simulink model "chap4_3sim"  (Simulink 8.3)
settings: Solver=ode45  StartTime=0.0  StopTime=10.0  RelTol=1e-3
libraries: fuzblock x1
settings Model: Creator=duan  LastModifiedBy=duan
settings DataIOCC: SignalLoggingSaveFormat=Dataset
settings DebuggingCC: UnderspecifiedInitializationDetection=Simplified  StateNameClashWarn=none
settings GRTTargetCC: CombineOutputUpdateFcns=on  GRTInterface=off

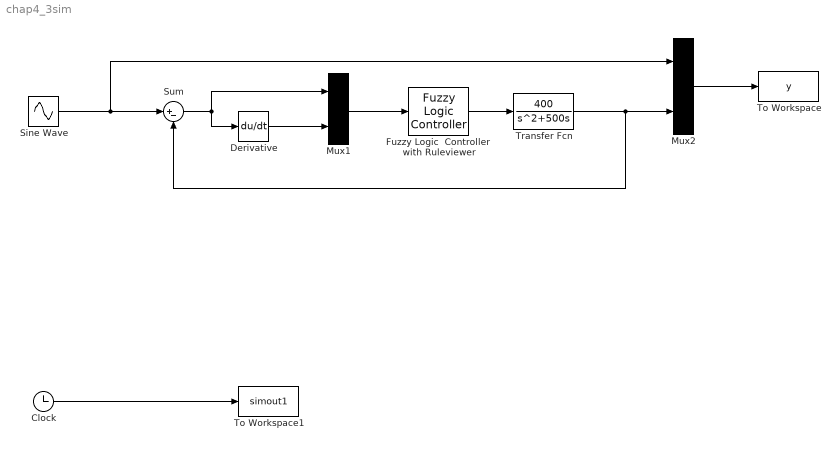
== system chap4_3sim ==
  Clock : Clock
  Derivative : Derivative
  Fuzzy Logic  Controller  with Ruleviewer : fuzblock/Fuzzy Logic  Controller  fis=[]
  Mux1 : Mux  Inputs=2
  Mux2 : Mux  Inputs=2
  Sine Wave : Sin  SampleTime=0
  Sum : Sum  Inputs=|+-
  To Workspace : ToWorkspace  VariableName=y  SaveFormat=Timeseries  SampleTime=-1
  To Workspace1 : ToWorkspace  VariableName=simout1  SaveFormat=Timeseries  SampleTime=-1
  Transfer Fcn : TransferFcn  Numerator=[400]  Denominator=[1 500 0]
  wires:
  Clock/1 -> To Workspace1/1
  Sine Wave/1 -> Mux2/1, Sum/1
  Sum/1 -> Derivative/1, Mux1/1
  Derivative/1 -> Mux1/2
  Mux1/1 -> Fuzzy Logic  Controller  with Ruleviewer/1
  Fuzzy Logic  Controller  with Ruleviewer/1 -> Transfer Fcn/1
  Transfer Fcn/1 -> Sum/2, Mux2/2
  Mux2/1 -> To Workspace/1
